simulink model "robot_sim_plant"  (R2025b)
settings: Solver=VariableStepAuto  StartTime=0.0  StopTime=10.0  RelTol=1e-3
values from neighbouring files (symbols this model uses):
  alpha = 1    [FIREFIGHTER_AID.m]    (also in Setup_CSDR_Simulation.m = -1.57079632679; Setup_CSDR_Simulation_NL.m = -1.57079632679)
  D = [d1 0; 0 d2]    [Setup_CSDR_Simulation.m]    (also in Setup_CSDR_Simulation_NL.m)
  g = 1    [FIREFIGHTER_AID.m]    (also in Setup_CSDR_Simulation.m = 9.81; Setup_CSDR_Simulation_NL.m = 9.81)
  I1 = 1.5    [Setup_CSDR_Simulation.m]    (also in Setup_CSDR_Simulation_NL.m)
  I2 = 0.5    [Setup_CSDR_Simulation.m]    (also in Setup_CSDR_Simulation_NL.m)
  Kd1 = 250    [Setup_CSDR_Simulation.m]
  Kd2 = 150    [Setup_CSDR_Simulation.m]
  Ki1 = 150    [Setup_CSDR_Simulation.m]
  Ki2 = 120    [Setup_CSDR_Simulation.m]
  Kp1 = 500    [Setup_CSDR_Simulation.m]
  Kp2 = 400    [Setup_CSDR_Simulation.m]
  l_c1 = 1    [FIREFIGHTER_AID.m]    (also in Setup_CSDR_Simulation.m = 0.5; Setup_CSDR_Simulation_NL.m = 0.5)
  m1 = 1    [FIREFIGHTER_AID.m]    (also in Setup_CSDR_Simulation.m = 15; Setup_CSDR_Simulation_NL.m = 15)
  m2 = 1    [FIREFIGHTER_AID.m]    (also in Setup_CSDR_Simulation.m = 8; Setup_CSDR_Simulation_NL.m = 8)
  S = eye(2)    [Setup_CSDR_Simulation.m]    (also in Setup_CSDR_Simulation_NL.m)
settings Model: Creator=sjoer  LastModifiedBy=sjoer

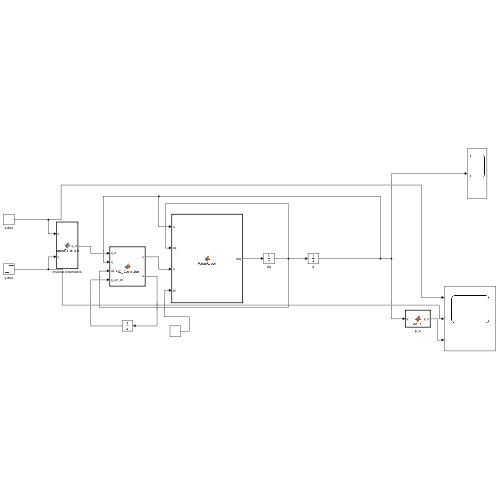
[thumbnail: Simulink's stored preview of the top-level diagram]
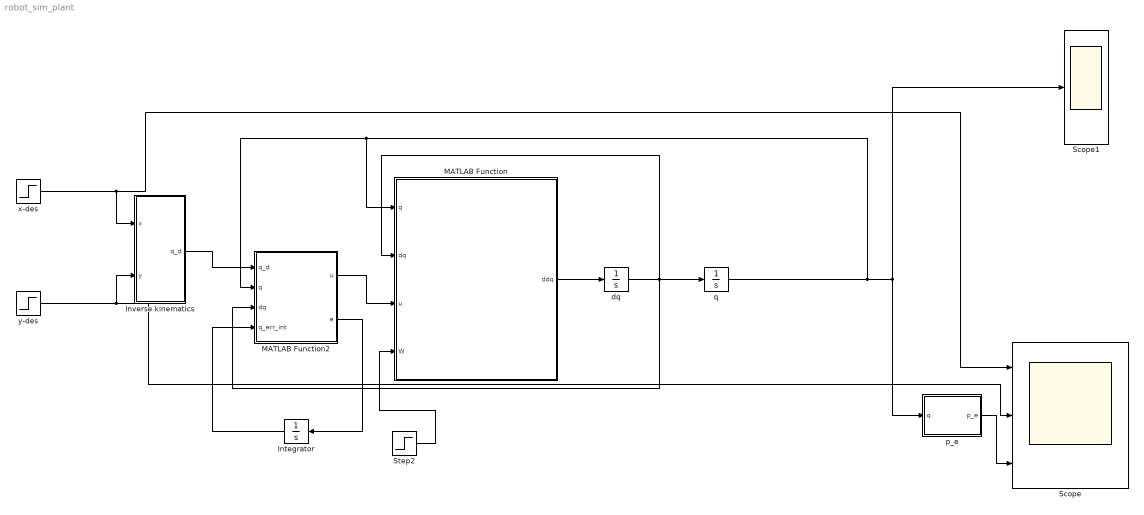
== system robot_sim_plant ==
  Integrator : Integrator
  Inverse kinematics : MATLAB Function  TreatAsAtomicUnit=on
  MATLAB Function : MATLAB Function  TreatAsAtomicUnit=on
  MATLAB Function2 : MATLAB Function  TreatAsAtomicUnit=on
  Scope : Scope  NumInputPorts=3
      settings: ActiveDisplayYMinimum=-2.4236587430684091  ActiveDisplayYMaximum=6.954835399262886
  Scope1 : Scope
      settings: ActiveDisplayYMinimum=-0.67574150627668172  ActiveDisplayYMaximum=2.283218801662231
  Step2 : Step  After=[0;0]  SampleTime=0
  dq : Integrator
  p_e : MATLAB Function  TreatAsAtomicUnit=on
  q : Integrator
  x-des : Step  Time=2  Before=3  After=4  SampleTime=0
  y-des : Step  Time=2  Before=3  After=4  SampleTime=0
  wires:
  MATLAB Function/1(ddq) -> dq/1
  q/1 -> MATLAB Function2/2(q), MATLAB Function/1(q), Scope1/1, p_e/1(q)
  Step2/1 -> MATLAB Function/4(W)
  p_e/1(p_e) -> Scope/3
  Inverse kinematics/1(q_d) -> MATLAB Function2/1(q_d)
  dq/1 -> MATLAB Function2/3(dq), q/1, MATLAB Function/2(dq)
  MATLAB Function2/2(e) -> Integrator/1
  Integrator/1 -> MATLAB Function2/4(q_err_int)
  MATLAB Function2/1(u) -> MATLAB Function/3(u)
  x-des/1 -> Scope/1, Inverse kinematics/1(x)
  y-des/1 -> Scope/2, Inverse kinematics/2(y)

== matlab function robot_sim_plant/p_e ==
  data: q input; p_e output
function p_e = ee_p(q)

p_e = [q(2)*cos(q(1)); q(2)*sin(q(1))];

== matlab function robot_sim_plant/MATLAB Function ==
  data: q input; ddq output; dq input; u input; W input; I1 parameter; I2 parameter; l_c1 parameter; m1 parameter; m2 parameter; S parameter; D parameter; g parameter; alpha parameter
function ddq  = PolarRobot(q, dq, u, W, I1, I2, l_c1, m1, m2, S, D, g, alpha)
% Only the dynamic equations remain here

% Vectors
q1 = q(1);
q2 = q(2);
dq_1 = dq(1);
dq_2 = dq(2);

% M(q) - Mass matrix (Changes with q2)
M = [I1 + I2 + (l_c1^2)*m1 + m2*(q2^2), 0;
     0, m2];

% c(q,dq) - Coriolis (Changes with q2, dq1, dq2)
c = [2*dq_1*dq_2*m2*q2;
    -(dq_1^2)*m2*q2];

% G(q) - Gravity (Changes with q1, q2)
G = [g*cos(alpha - q1)*(l_c1*m1 + m2*q2);
    -g*m2*sin(alpha - q1)];

% J(q) - Jacobian
J = [-q2*sin(q1), cos(q1);
      q2*cos(q1), sin(q1)];

% Solving for ddq
ddq = M \ (S*u + J'* W - c - D*dq - G);

== matlab function robot_sim_plant/Inverse kinematics ==
  data: x input; q_d output size=2 1; y input
function q_d  = InverseKinematics(x, y)
    % This block runs every time step
    
    % Extension (Prismatic Joint)
    q2_d = sqrt(x^2 + y^2);
    
    % Rotation (Revolute Joint)
    % We use atan2 to handle all quadrants automatically
    q1_d = atan2(y, x);

    q_d = [q1_d; q2_d];
end

== matlab function robot_sim_plant/MATLAB Function2 ==
  data: q_d input size=2 1; u output size=2 1; q input size=2 1; dq input; q_err_int input; Kp1 parameter; Ki1 parameter; Kd1 parameter; Kp2 parameter; Ki2 parameter; Kd2 parameter; e output size=2 1
function [u, e] = PID_Controller(q_d, q, dq, q_err_int, Kp1, Ki1, Kd1, Kp2, Ki2, Kd2)
% q_d       : Desired [q1; q2]
% q         : Actual  [q1; q2]
% dq_d      : Desired velocity [0; 0]
% dq        : Actual velocity [dq1; dq2]
% q_err_int : Integrated error from external Simulink Integrator

% 1. Internal Error Calculation
e = q_d - q;


% 2. PID Law
% Joint 1 (Rotation)
tau = (Kp1 * e(1)) + (Ki1 * q_err_int(1)) - (Kd1 * dq(1));

% Joint 2 (Prismatic)
F   = (Kp2 * e(2)) + (Ki2 * q_err_int(2)) - (Kd2 * dq(2));

u = [tau; F];

end
